simulink model "sampleModel7424_pp"  (R2018a)
settings: Solver=VariableStepAuto  StartTime=0.0  StopTime=10.0  RelTol=1e-3
undefined symbols (not defined in the file): DiscIntNeverNeededParam
libraries: simulink x211
(part 3 of 5)

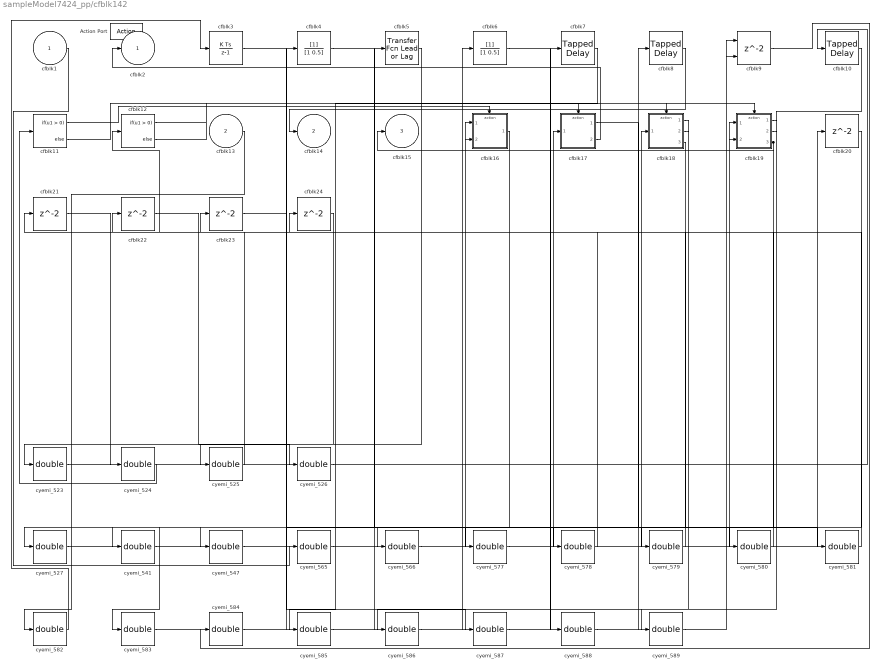
== system sampleModel7424_pp/cfblk142 ==
  cfblk1 : Inport
  cfblk13 : Inport  Port=2
  Action Port : ActionPort  ActionType=else
  cfblk10 : simulink/Discrete/Tapped Delay  vinit=0.0  samptime=-1  NumDelays=1  DelayOrder=Oldest  includeCurrent=off
  cfblk11 : If  SampleTime=1
  cfblk12 : If  SampleTime=1
  cfblk16 : Subsystem  TreatAsAtomicUnit=on
  cfblk17 : Subsystem  TreatAsAtomicUnit=on
  cfblk18 : Subsystem  TreatAsAtomicUnit=on
  cfblk19 : Subsystem  TreatAsAtomicUnit=on
  cfblk{20..24} (5 alike) : Delay
  cfblk3 : DiscreteIntegrator  SampleTime=-1  OutDataTypeStr=double  ICPrevOutput=DiscIntNeverNeededParam  ICPrevScaledInput=DiscIntNeverNeededParam
  cfblk4 : DiscreteFilter
  cfblk5 : simulink/Discrete/Transfer Fcn Lead or Lag  PoleZ=0.95  ZeroZ=0.75  ICPrevOutput=0.0  ICPrevInput=0.0  DoSatur=off
      settings: SourceProductName=Simulink  SourceProductBaseCode=SL
  cfblk6 : DiscreteFilter
  cfblk7 : simulink/Discrete/Tapped Delay  vinit=0.0  samptime=-1  NumDelays=1  DelayOrder=Oldest  includeCurrent=off
  cfblk8 : simulink/Discrete/Tapped Delay  vinit=0.0  samptime=-1  NumDelays=1  DelayOrder=Oldest  includeCurrent=off
  cfblk9 : Delay  ShowEnablePort=on
      settings: InputPortMap=u0,e6
  cyemi_{523..527,541,547,565..566,577..589} (22 alike) : DataTypeConversion  OutDataTypeStr=double
  cfblk2 : Outport
  cfblk14 : Outport  Port=2
  cfblk15 : Outport  Port=3
  wires:
  cfblk8/1 -> cfblk14/1
  cfblk19/3(cfblk13) -> cfblk15/1, cyemi_582/1
  cfblk17/2(cfblk7) -> cfblk2/1
  cfblk11/1 -> cfblk16/Action
  cfblk11/2 -> cfblk17/Action
  cfblk12/1 -> cfblk18/Action
  cfblk12/2 -> cfblk19/Action
  cyemi_523/1 -> cfblk10/1
  cfblk5/1 -> cyemi_523/1
  cyemi_524/1 -> cfblk11/1
  cfblk21/1 -> cyemi_524/1
  cyemi_525/1 -> cfblk12/1
  cfblk24/1 -> cyemi_525/1
  cyemi_526/1 -> cfblk16/1(cfblk1)
  cfblk22/1 -> cyemi_526/1
  cyemi_527/1 -> cfblk16/2(cfblk11)
  cfblk13/1 -> cyemi_527/1
  cyemi_541/1 -> cfblk17/1(cfblk1)
  cfblk19/1(cfblk2) -> cyemi_541/1
  cyemi_547/1 -> cfblk18/1(cfblk1)
  cfblk20/1 -> cyemi_547/1
  cyemi_565/1 -> cfblk19/1(cfblk1)
  cfblk1/1 -> cyemi_565/1
  cyemi_566/1 -> cfblk19/2(cfblk11)
  cfblk23/1 -> cyemi_566/1
  cyemi_577/1 -> cfblk20/1
  cfblk16/1(cfblk2) -> cyemi_577/1
  cyemi_578/1 -> cfblk21/1
  cfblk10/1 -> cyemi_578/1
  cyemi_579/1 -> cfblk22/1
  cfblk18/2(cfblk14) -> cyemi_579/1
  cyemi_580/1 -> cfblk23/1
  cfblk4/1 -> cyemi_580/1
  cyemi_581/1 -> cfblk24/1
  cfblk17/1(cfblk2) -> cyemi_581/1
  cyemi_582/1 -> cfblk3/1
  cyemi_583/1 -> cfblk4/1
  cfblk18/3(cfblk15) -> cyemi_583/1
  cyemi_584/1 -> cfblk5/1
  cfblk9/1 -> cyemi_584/1
  cyemi_585/1 -> cfblk6/1
  cfblk7/1 -> cyemi_585/1
  cyemi_586/1 -> cfblk7/1
  cfblk19/2(cfblk12) -> cyemi_586/1
  cyemi_587/1 -> cfblk8/1
  cfblk3/1 -> cyemi_587/1
  cyemi_588/1 -> cfblk9/1
  cfblk6/1 -> cyemi_588/1
  cyemi_589/1 -> cfblk9/2
  cfblk18/1(cfblk2) -> cyemi_589/1

== system sampleModel7424_pp/cfblk143 ==
  cfblk1 : Inport
  Action Port : ActionPort  ActionType=then
  cfblk3 : UnitDelay  SampleTime=-1
  cfblk4 : DiscreteZeroPole  Poles=[0 0.5]  Gain=1  SampleTime=-1
  cfblk5 : DiscreteZeroPole  Poles=[0 0.5]  Gain=1  SampleTime=-1
  cfblk6 : simulink/Discrete/Transfer Fcn First Order  PoleZ=0.95  ICPrevOutput=0.0  DoSatur=off
      settings: SourceProductName=Simulink
  cfblk7 : DiscreteZeroPole  Poles=[0 0.5]  Gain=1  SampleTime=-1
  cfblk8 : Delay
  cfblk9 : DataTypeConversion  OutDataTypeStr=double
  cyemi_{591..596} (6 alike) : DataTypeConversion  OutDataTypeStr=double
  cyemi_597 : DataTypeConversion  OutDataTypeStr=uint16
  cfblk2 : Outport
  wires:
  cfblk7/1 -> cfblk2/1
  cyemi_591/1 -> cfblk3/1
  cfblk8/1 -> cyemi_591/1
  cyemi_592/1 -> cfblk4/1
  cfblk6/1 -> cyemi_592/1
  cyemi_593/1 -> cfblk5/1
  cfblk4/1 -> cyemi_593/1
  cyemi_594/1 -> cfblk6/1
  cfblk3/1 -> cyemi_594/1
  cyemi_595/1 -> cfblk7/1
  cfblk9/1 -> cyemi_595/1
  cyemi_596/1 -> cfblk8/1
  cfblk5/1 -> cyemi_596/1
  cyemi_597/1 -> cfblk9/1
  cfblk1/1 -> cyemi_597/1

== system sampleModel7424_pp/cfblk144 ==
  cfblk1 : Inport
  cfblk12 : Inport  Port=2
  cfblk13 : Inport  Port=3
  Action Port : ActionPort  ActionType=else
  cfblk10 : simulink/Continuous/PID Controller  Controller=PID  TimeDomain=Discrete-time  SampleTime=-1  IntegratorMethod=Forward Euler  FilterMethod=Forward Euler  Form=Parallel  UseFilter=on  ControllerParametersSource=internal  P=1  I=1  D=0  N=100  InitialConditionSource=internal  InitialConditionForIntegrator=0  InitialConditionForFilter=0  ExternalReset=none  LimitOutput=off  UpperSaturationLimit=inf  LowerSaturationLimit=-inf  LinearizeAsGain=off  AntiWindupMode=none  Kb=1  TrackingMode=off  Kt=1  PParamMin=[]  PParamMax=[]  IParamMin=[]  IParamMax=[]  DParamMin=[]  DParamMax=[]  NParamMin=[]  NParamMax=[]  KbParamMin=[]  KbParamMax=[]  KtParamMin=[]  KtParamMax=[]  POutMin=[]  POutMax=[]  IOutMin=[]  IOutMax=[]  DOutMin=[]  DOutMax=[]  NOutMin=[]  NOutMax=[]  KbOutMin=[]  KbOutMax=[]  KtOutMin=[]  KtOutMax=[]  IntegratorOutMin=[]  IntegratorOutMax=[]  FilterOutMin=[]  FilterOutMax=[]  SumOutMin=[]  SumOutMax=[]  SumI1OutMin=[]  SumI1OutMax=[]  SumI2OutMin=[]  SumI2OutMax=[]  SumI3OutMin=[]  SumI3OutMax=[]  SumDOutMin=[]  SumDOutMax=[]  SaturationOutMin=[]  SaturationOutMax=[]  IntegratorContinuousStateAttributes=''  IntegratorStateMustResolveToSignalObject=off  IntegratorRTWStateStorageClass=Auto  FilterContinuousStateAttributes=''  FilterStateMustResolveToSignalObject=off  FilterRTWStateStorageClass=Auto  DifferentiatorICPrevScaledInput=0  DifferentiatorOutMin=[]  DifferentiatorOutMax=[]  FilterDiffOutCoefMin=[]  FilterDiffOutCoefMax=[]  SumDenOutMin=[]  SumDenOutMax=[]  SumNumOutMin=[]  SumNumOutMax=[]  ReciprocalOutMin=[]  ReciprocalOutMax=[]  DivideOutMin=[]  DivideOutMax=[]  TunerSelectOption=Transfer Function Based (PID Tuner App)
  cfblk11 : Delay  DelayLengthSource=Input port
      settings: InputPortMap=u0,p1
  cfblk14 : Delay
  cfblk3 : simulink/Discrete/Tapped Delay  vinit=0.0  samptime=-1  NumDelays=1  DelayOrder=Oldest  includeCurrent=off
  cfblk4 : simulink/Continuous/PID Controller  Controller=PID  TimeDomain=Discrete-time  SampleTime=-1  IntegratorMethod=Forward Euler  FilterMethod=Forward Euler  Form=Parallel  UseFilter=on  ControllerParametersSource=internal  P=1  I=1  D=0  N=100  InitialConditionSource=internal  InitialConditionForIntegrator=0  InitialConditionForFilter=0  ExternalReset=none  LimitOutput=off  UpperSaturationLimit=inf  LowerSaturationLimit=-inf  LinearizeAsGain=off  AntiWindupMode=none  Kb=1  TrackingMode=off  Kt=1  PParamMin=[]  PParamMax=[]  IParamMin=[]  IParamMax=[]  DParamMin=[]  DParamMax=[]  NParamMin=[]  NParamMax=[]  KbParamMin=[]  KbParamMax=[]  KtParamMin=[]  KtParamMax=[]  POutMin=[]  POutMax=[]  IOutMin=[]  IOutMax=[]  DOutMin=[]  DOutMax=[]  NOutMin=[]  NOutMax=[]  KbOutMin=[]  KbOutMax=[]  KtOutMin=[]  KtOutMax=[]  IntegratorOutMin=[]  IntegratorOutMax=[]  FilterOutMin=[]  FilterOutMax=[]  SumOutMin=[]  SumOutMax=[]  SumI1OutMin=[]  SumI1OutMax=[]  SumI2OutMin=[]  SumI2OutMax=[]  SumI3OutMin=[]  SumI3OutMax=[]  SumDOutMin=[]  SumDOutMax=[]  SaturationOutMin=[]  SaturationOutMax=[]  IntegratorContinuousStateAttributes=''  IntegratorStateMustResolveToSignalObject=off  IntegratorRTWStateStorageClass=Auto  FilterContinuousStateAttributes=''  FilterStateMustResolveToSignalObject=off  FilterRTWStateStorageClass=Auto  DifferentiatorICPrevScaledInput=0  DifferentiatorOutMin=[]  DifferentiatorOutMax=[]  FilterDiffOutCoefMin=[]  FilterDiffOutCoefMax=[]  SumDenOutMin=[]  SumDenOutMax=[]  SumNumOutMin=[]  SumNumOutMax=[]  ReciprocalOutMin=[]  ReciprocalOutMax=[]  DivideOutMin=[]  DivideOutMax=[]  TunerSelectOption=Transfer Function Based (PID Tuner App)
  cfblk5 : simulink/Discrete/Transfer Fcn Real Zero  ZeroZ=0.75  ICPrevInput=0.0  DoSatur=off
      settings: SourceProductName=Simulink  SourceProductBaseCode=SL
  cfblk6 : DiscreteFir
  cfblk7 : DiscreteFir
  cfblk8 : DiscreteTransferFcn
  cfblk9 : simulink/Discrete/Transfer Fcn Lead or Lag  PoleZ=0.95  ZeroZ=0.75  ICPrevOutput=0.0  ICPrevInput=0.0  DoSatur=off
      settings: SourceProductName=Simulink  SourceProductBaseCode=SL
  cyemi_{601..611} (11 alike) : DataTypeConversion  OutDataTypeStr=double
  cfblk2 : Outport
  wires:
  cfblk12/1 -> cfblk2/1
  cyemi_601/1 -> cfblk10/1
  cfblk5/1 -> cyemi_601/1
  cyemi_602/1 -> cfblk11/1
  cfblk1/1 -> cyemi_602/1
  cyemi_603/1 -> cfblk11/2
  cfblk3/1 -> cyemi_603/1
  cyemi_604/1 -> cfblk14/1
  cfblk7/1 -> cyemi_604/1
  cyemi_605/1 -> cfblk3/1
  cfblk9/1 -> cyemi_605/1
  cyemi_606/1 -> cfblk4/1
  cfblk13/1 -> cyemi_606/1
  cyemi_607/1 -> cfblk5/1
  cfblk4/1 -> cyemi_607/1
  cyemi_608/1 -> cfblk6/1
  cfblk14/1 -> cyemi_608/1
  cyemi_609/1 -> cfblk7/1
  cfblk8/1 -> cyemi_609/1
  cyemi_610/1 -> cfblk8/1
  cfblk6/1 -> cyemi_610/1
  cyemi_611/1 -> cfblk9/1
  cfblk10/1 -> cyemi_611/1

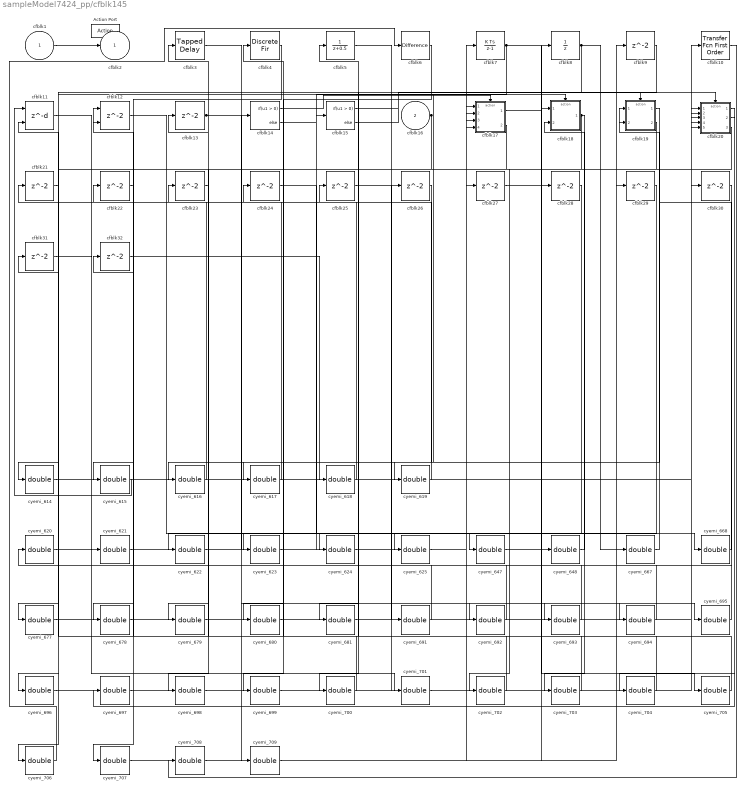
== system sampleModel7424_pp/cfblk145 ==
  cfblk1 : Inport
  cfblk16 : Inport  Port=2
  Action Port : ActionPort  ActionType=then
  cfblk10 : simulink/Discrete/Transfer Fcn First Order  PoleZ=0.95  ICPrevOutput=0.0  DoSatur=off
      settings: SourceProductName=Simulink
  cfblk11 : Delay  DelayLengthSource=Input port
      settings: InputPortMap=u0,p1
  cfblk12 : Delay  ShowEnablePort=on
      settings: InputPortMap=u0,e6
  cfblk{9,13,21..32} (14 alike) : Delay
  cfblk14 : If  SampleTime=1
  cfblk15 : If  SampleTime=1
  cfblk17 : Subsystem  TreatAsAtomicUnit=on
  cfblk18 : Subsystem  TreatAsAtomicUnit=on
  cfblk19 : Subsystem  TreatAsAtomicUnit=on
  cfblk20 : Subsystem  TreatAsAtomicUnit=on
  cfblk3 : simulink/Discrete/Tapped Delay  vinit=0.0  samptime=-1  NumDelays=1  DelayOrder=Oldest  includeCurrent=off
  cfblk4 : DiscreteFir
  cfblk5 : DiscreteTransferFcn
  cfblk6 : simulink/Discrete/Difference  ICPrevInput=0.0  OutMin=[]  OutMax=[]  OutDataTypeStr=double  OutputDataTypeScalingMode=double  OutDataType=fixdt(1, 16)  OutScaling=2^-10  DoSatur=off
  cfblk7 : DiscreteIntegrator  SampleTime=-1  OutDataTypeStr=double  ICPrevOutput=DiscIntNeverNeededParam  ICPrevScaledInput=DiscIntNeverNeededParam
  cfblk8 : UnitDelay  SampleTime=-1
  cyemi_{614..625,647..648,667..668,677..681,691..709} (40 alike) : DataTypeConversion  OutDataTypeStr=double
  cfblk2 : Outport
  wires:
  cfblk1/1 -> cfblk2/1
  cfblk8/1 -> cyemi_667/1, cyemi_681/1
  cfblk16/1 -> cyemi_615/1, cyemi_680/1
  cfblk13/1 -> cyemi_692/1, cyemi_693/1, cyemi_694/1
  cfblk7/1 -> cyemi_619/1, cyemi_695/1, cyemi_696/1
  cfblk18/1(cfblk2) -> cyemi_614/1, cyemi_624/1, cyemi_703/1
  cfblk14/1 -> cfblk17/Action
  cfblk14/2 -> cfblk18/Action
  cfblk15/1 -> cfblk19/Action
  cfblk15/2 -> cfblk20/Action
  cyemi_614/1 -> cfblk10/1
  cyemi_615/1 -> cfblk11/1
  cyemi_616/1 -> cfblk11/2
  cfblk19/1(cfblk2) -> cyemi_616/1
  cyemi_617/1 -> cfblk12/1
  cfblk6/1 -> cyemi_617/1
  cyemi_618/1 -> cfblk12/2
  cfblk32/1 -> cyemi_618/1
  cyemi_619/1 -> cfblk13/1
  cyemi_620/1 -> cfblk14/1
  cfblk30/1 -> cyemi_620/1
  cyemi_621/1 -> cfblk15/1
  cfblk31/1 -> cyemi_621/1
  cyemi_622/1 -> cfblk17/1(cfblk1)
  cfblk28/1 -> cyemi_622/1
  cyemi_623/1 -> cfblk17/2(cfblk14)
  cfblk26/1 -> cyemi_623/1
  cyemi_624/1 -> cfblk17/3(cfblk15)
  cyemi_625/1 -> cfblk17/4(cfblk16)
  cfblk24/1 -> cyemi_625/1
  cyemi_647/1 -> cfblk18/1(cfblk1)
  cfblk12/1 -> cyemi_647/1
  cyemi_648/1 -> cfblk18/2(cfblk15)
  cfblk27/1 -> cyemi_648/1
  cyemi_667/1 -> cfblk19/1(cfblk1)
  cyemi_668/1 -> cfblk19/2(cfblk11)
  cfblk25/1 -> cyemi_668/1
  cyemi_677/1 -> cfblk20/1(cfblk1)
  cfblk21/1 -> cyemi_677/1
  cyemi_678/1 -> cfblk20/2(cfblk10)
  cfblk22/1 -> cyemi_678/1
  cyemi_679/1 -> cfblk20/3(cfblk11)
  cfblk23/1 -> cyemi_679/1
  cyemi_680/1 -> cfblk20/4(cfblk12)
  cyemi_681/1 -> cfblk20/5(cfblk13)
  cyemi_691/1 -> cfblk21/1
  cfblk5/1 -> cyemi_691/1
  cyemi_692/1 -> cfblk22/1
  cyemi_693/1 -> cfblk23/1
  cyemi_694/1 -> cfblk24/1
  cyemi_695/1 -> cfblk25/1
  cyemi_696/1 -> cfblk26/1
  cyemi_697/1 -> cfblk27/1
  cfblk20/2(cfblk14) -> cyemi_697/1
  cyemi_698/1 -> cfblk28/1
  cfblk20/3(cfblk15) -> cyemi_698/1
  cyemi_699/1 -> cfblk29/1
  cfblk17/2(cfblk17) -> cyemi_699/1
  cyemi_700/1 -> cfblk3/1
  cfblk29/1 -> cyemi_700/1
  cyemi_701/1 -> cfblk30/1
  cfblk11/1 -> cyemi_701/1
  cyemi_702/1 -> cfblk31/1
  cfblk19/2(cfblk12) -> cyemi_702/1
  cyemi_703/1 -> cfblk32/1
  cyemi_704/1 -> cfblk4/1
  cfblk20/1(cfblk2) -> cyemi_704/1
  cyemi_705/1 -> cfblk5/1
  cfblk17/1(cfblk2) -> cyemi_705/1
  cyemi_706/1 -> cfblk6/1
  cfblk9/1 -> cyemi_706/1
  cyemi_707/1 -> cfblk7/1
  cfblk4/1 -> cyemi_707/1
  cyemi_708/1 -> cfblk8/1
  cfblk10/1 -> cyemi_708/1
  cyemi_709/1 -> cfblk9/1
  cfblk3/1 -> cyemi_709/1

== system sampleModel7424_pp/cfblk146 ==
  cfblk1 : Inport
  cfblk10 : Inport  Port=2
  Action Port : ActionPort  ActionType=else
  cfblk3 : UnitDelay  SampleTime=-1
  cfblk4 : DiscreteFilter
  cfblk5 : DiscreteZeroPole  Poles=[0 0.5]  Gain=1  SampleTime=-1
  cfblk6 : simulink/Discrete/Difference  ICPrevInput=0.0  OutMin=[]  OutMax=[]  OutDataTypeStr=double  OutputDataTypeScalingMode=double  OutDataType=fixdt(1, 16)  OutScaling=2^-10  DoSatur=off
  cfblk7 : simulink/Discrete/Difference  ICPrevInput=0.0  OutMin=[]  OutMax=[]  OutDataTypeStr=double  OutputDataTypeScalingMode=double  OutDataType=fixdt(1, 16)  OutScaling=2^-10  DoSatur=off
  cfblk8 : DiscreteFir
  cfblk9 : simulink/Continuous/PID Controller (2DOF)  Controller=PID  TimeDomain=Discrete-time  SampleTime=-1  IntegratorMethod=Forward Euler  FilterMethod=Forward Euler  Form=Parallel  UseFilter=on  ControllerParametersSource=internal  P=1  I=1  D=0  N=100  b=1  c=1  InitialConditionSource=internal  InitialConditionForIntegrator=0  InitialConditionForFilter=0  ExternalReset=none  LimitOutput=off  UpperSaturationLimit=inf  LowerSaturationLimit=-inf  LinearizeAsGain=off  AntiWindupMode=none  Kb=1  TrackingMode=off  Kt=1  PParamMin=[]  PParamMax=[]  IParamMin=[]  IParamMax=[]  DParamMin=[]  DParamMax=[]  NParamMin=[]  NParamMax=[]  bParamMin=[]  bParamMax=[]  cParamMin=[]  cParamMax=[]  KbParamMin=[]  KbParamMax=[]  KtParamMin=[]  KtParamMax=[]  POutMin=[]  POutMax=[]  IOutMin=[]  IOutMax=[]  DOutMin=[]  DOutMax=[]  NOutMin=[]  NOutMax=[]  bOutMin=[]  bOutMax=[]  cOutMin=[]  cOutMax=[]  KbOutMin=[]  KbOutMax=[]  KtOutMin=[]  KtOutMax=[]  IntegratorOutMin=[]  IntegratorOutMax=[]  FilterOutMin=[]  FilterOutMax=[]  SumOutMin=[]  SumOutMax=[]  Sum1OutMin=[]  Sum1OutMax=[]  Sum2OutMin=[]  Sum2OutMax=[]  Sum3OutMin=[]  Sum3OutMax=[]  SumI1OutMin=[]  SumI1OutMax=[]  SumI2OutMin=[]  SumI2OutMax=[]  SumI3OutMin=[]  SumI3OutMax=[]  SumDOutMin=[]  SumDOutMax=[]  SaturationOutMin=[]  SaturationOutMax=[]  IntegratorContinuousStateAttributes=''  IntegratorStateMustResolveToSignalObject=off  IntegratorRTWStateStorageClass=Auto  FilterContinuousStateAttributes=''  FilterStateMustResolveToSignalObject=off  FilterRTWStateStorageClass=Auto  DifferentiatorICPrevScaledInput=0  DifferentiatorOutMin=[]  DifferentiatorOutMax=[]  FilterDiffOutCoefMin=[]  FilterDiffOutCoefMax=[]  SumDenOutMin=[]  SumDenOutMax=[]  SumNumOutMin=[]  SumNumOutMax=[]  ReciprocalOutMin=[]  ReciprocalOutMax=[]  DivideOutMin=[]  DivideOutMax=[]  TunerSelectOption=Transfer Function Based (PID Tuner App)
  cyemi_{712..719} (8 alike) : DataTypeConversion  OutDataTypeStr=double
  cfblk2 : Outport
  cfblk11 : Outport  Port=2
  cfblk12 : Outport  Port=3
  wires:
  cfblk8/1 -> cfblk2/1
  cfblk4/1 -> cyemi_714/1, cyemi_719/1
  cfblk9/1 -> cfblk11/1
  cfblk6/1 -> cfblk12/1
  cfblk5/1 -> cyemi_712/1, cyemi_718/1
  cyemi_712/1 -> cfblk3/1
  cyemi_713/1 -> cfblk4/1
  cfblk10/1 -> cyemi_713/1
  cyemi_714/1 -> cfblk5/1
  cyemi_715/1 -> cfblk6/1
  cfblk7/1 -> cyemi_715/1
  cyemi_716/1 -> cfblk7/1
  cfblk3/1 -> cyemi_716/1
  cyemi_717/1 -> cfblk8/1
  cfblk1/1 -> cyemi_717/1
  cyemi_718/1 -> cfblk9/1
  cyemi_719/1 -> cfblk9/2

== system sampleModel7424_pp/cfblk147 ==
  cfblk1 : Inport
  cfblk10 : Inport  Port=2
  cfblk11 : Inport  Port=3
  Action Port : ActionPort  ActionType=then
  cfblk13 : Delay
  cfblk3 : DiscreteZeroPole  Poles=[0 0.5]  Gain=1  SampleTime=-1
  cfblk4 : Delay  DelayLengthSource=Input port
      settings: InputPortMap=u0,p1
  cfblk5 : DiscreteFilter
  cfblk6 : simulink/Discrete/Transfer Fcn First Order  PoleZ=0.95  ICPrevOutput=0.0  DoSatur=off
      settings: SourceProductName=Simulink
  cfblk7 : DiscreteFilter
  cfblk8 : DiscreteFilter
  cfblk9 : simulink/Discrete/Transfer Fcn Lead or Lag  PoleZ=0.95  ZeroZ=0.75  ICPrevOutput=0.0  ICPrevInput=0.0  DoSatur=off
      settings: SourceProductName=Simulink  SourceProductBaseCode=SL
  cyemi_{723..731} (9 alike) : DataTypeConversion  OutDataTypeStr=double
  cfblk2 : Outport
  cfblk12 : Outport  Port=2
  wires:
  cfblk3/1 -> cfblk2/1
  cfblk7/1 -> cfblk12/1
  cyemi_723/1 -> cfblk13/1
  cfblk8/1 -> cyemi_723/1
  cyemi_724/1 -> cfblk3/1
  cfblk5/1 -> cyemi_724/1
  cyemi_725/1 -> cfblk4/1
  cfblk13/1 -> cyemi_725/1
  cyemi_726/1 -> cfblk4/2
  cfblk9/1 -> cyemi_726/1
  cyemi_727/1 -> cfblk5/1
  cfblk10/1 -> cyemi_727/1
  cyemi_728/1 -> cfblk6/1
  cfblk4/1 -> cyemi_728/1
  cyemi_729/1 -> cfblk7/1
  cfblk11/1 -> cyemi_729/1
  cyemi_730/1 -> cfblk8/1
  cfblk6/1 -> cyemi_730/1
  cyemi_731/1 -> cfblk9/1
  cfblk1/1 -> cyemi_731/1

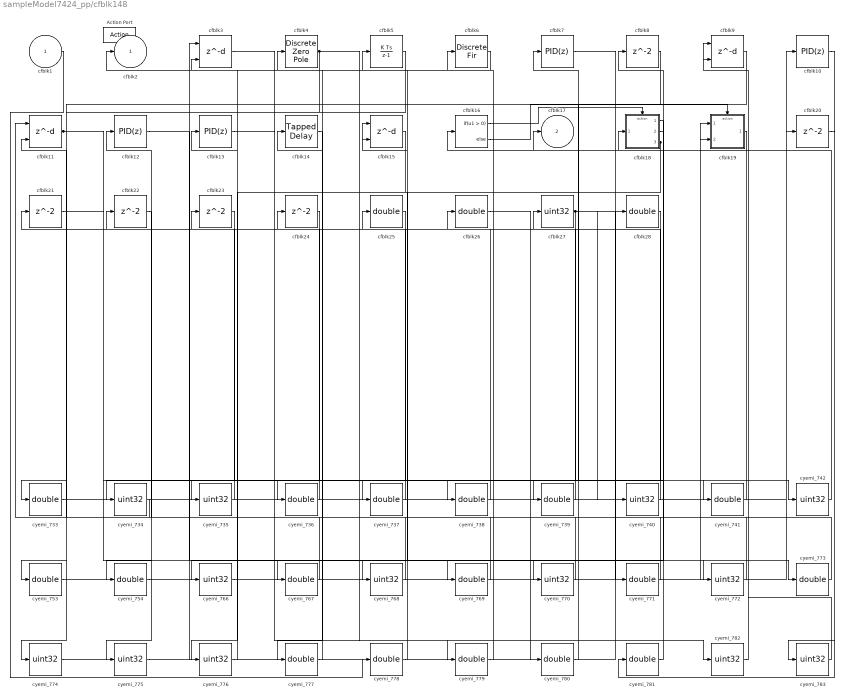
== system sampleModel7424_pp/cfblk148 ==
  cfblk1 : Inport
  Action Port : ActionPort  ActionType=else
  cfblk{7,10,12..13} (4 alike) : simulink/Continuous/PID Controller  Controller=PID  TimeDomain=Discrete-time  SampleTime=-1  IntegratorMethod=Forward Euler  FilterMethod=Forward Euler  Form=Parallel  UseFilter=on  ControllerParametersSource=internal  P=1  I=1  D=0  N=100  InitialConditionSource=internal  InitialConditionForIntegrator=0  InitialConditionForFilter=0  ExternalReset=none  LimitOutput=off  UpperSaturationLimit=inf  LowerSaturationLimit=-inf  LinearizeAsGain=off  AntiWindupMode=none  Kb=1  TrackingMode=off  Kt=1  PParamMin=[]  PParamMax=[]  IParamMin=[]  IParamMax=[]  DParamMin=[]  DParamMax=[]  NParamMin=[]  NParamMax=[]  KbParamMin=[]  KbParamMax=[]  KtParamMin=[]  KtParamMax=[]  POutMin=[]  POutMax=[]  IOutMin=[]  IOutMax=[]  DOutMin=[]  DOutMax=[]  NOutMin=[]  NOutMax=[]  KbOutMin=[]  KbOutMax=[]  KtOutMin=[]  KtOutMax=[]  IntegratorOutMin=[]  IntegratorOutMax=[]  FilterOutMin=[]  FilterOutMax=[]  SumOutMin=[]  SumOutMax=[]  SumI1OutMin=[]  SumI1OutMax=[]  SumI2OutMin=[]  SumI2OutMax=[]  SumI3OutMin=[]  SumI3OutMax=[]  SumDOutMin=[]  SumDOutMax=[]  SaturationOutMin=[]  SaturationOutMax=[]  IntegratorContinuousStateAttributes=''  IntegratorStateMustResolveToSignalObject=off  IntegratorRTWStateStorageClass=Auto  FilterContinuousStateAttributes=''  FilterStateMustResolveToSignalObject=off  FilterRTWStateStorageClass=Auto  DifferentiatorICPrevScaledInput=0  DifferentiatorOutMin=[]  DifferentiatorOutMax=[]  FilterDiffOutCoefMin=[]  FilterDiffOutCoefMax=[]  SumDenOutMin=[]  SumDenOutMax=[]  SumNumOutMin=[]  SumNumOutMax=[]  ReciprocalOutMin=[]  ReciprocalOutMax=[]  DivideOutMin=[]  DivideOutMax=[]  TunerSelectOption=Transfer Function Based (PID Tuner App)
  cfblk{3,9,11,15} (4 alike) : Delay  DelayLengthSource=Input port
      settings: InputPortMap=u0,p1
  cfblk14 : simulink/Discrete/Tapped Delay  vinit=0.0  samptime=-1  NumDelays=1  DelayOrder=Oldest  includeCurrent=off
  cfblk16 : If  SampleTime=1
  cfblk18 : Subsystem  TreatAsAtomicUnit=on
  cfblk19 : Subsystem  TreatAsAtomicUnit=on
  cfblk{8,20..24} (6 alike) : Delay
  cfblk25 : DataTypeConversion  OutDataTypeStr=double
  cfblk26 : DataTypeConversion  OutDataTypeStr=double
  cfblk27 : DataTypeConversion  OutDataTypeStr=uint32
  cfblk28 : DataTypeConversion  OutDataTypeStr=double
  cfblk4 : DiscreteZeroPole  Poles=[0 0.5]  Gain=1  SampleTime=-1
  cfblk5 : DiscreteIntegrator  SampleTime=-1  OutDataTypeStr=double  ICPrevOutput=DiscIntNeverNeededParam  ICPrevScaledInput=DiscIntNeverNeededParam
  cfblk6 : DiscreteFir
  cyemi_{733,736..739,741,753..754,767,769,771,773,777..781} (17 alike) : DataTypeConversion  OutDataTypeStr=double
  cyemi_{734..735,740,742,766,768,770,772,774..776,782..783} (13 alike) : DataTypeConversion  OutDataTypeStr=uint32
  cfblk2 : Outport
  cfblk17 : Outport  Port=2
  wires:
  cfblk4/1 -> cyemi_753/1, cyemi_779/1
  cfblk11/1 -> cyemi_770/1, cyemi_772/1
  cfblk6/1 -> cfblk2/1
  cfblk19/1(cfblk2) -> cfblk17/1
  cfblk18/3(cfblk10) -> cyemi_735/1, cyemi_768/1
  cfblk16/1 -> cfblk18/Action
  cfblk16/2 -> cfblk19/Action
  cfblk27/1 -> cyemi_734/1, cyemi_740/1, cyemi_742/1
  cyemi_733/1 -> cfblk10/1
  cfblk5/1 -> cyemi_733/1
  cyemi_734/1 -> cfblk11/1
  cyemi_735/1 -> cfblk11/2
  cyemi_736/1 -> cfblk12/1
  cfblk25/1 -> cyemi_736/1
  cyemi_737/1 -> cfblk13/1
  cfblk28/1 -> cyemi_737/1
  cyemi_738/1 -> cfblk14/1
  cfblk18/2(cfblk9) -> cyemi_738/1
  cyemi_739/1 -> cfblk15/1
  cfblk8/1 -> cyemi_739/1
  cyemi_740/1 -> cfblk15/2
  cyemi_741/1 -> cfblk16/1
  cfblk21/1 -> cyemi_741/1
  cyemi_742/1 -> cfblk18/1(cfblk1)
  cyemi_753/1 -> cfblk19/1(cfblk1)
  cyemi_754/1 -> cfblk19/2(cfblk11)
  cfblk23/1 -> cyemi_754/1
  cyemi_766/1 -> cfblk20/1
  cfblk18/1(cfblk2) -> cyemi_766/1
  cyemi_767/1 -> cfblk21/1
  cfblk14/1 -> cyemi_767/1
  cyemi_768/1 -> cfblk22/1
  cyemi_769/1 -> cfblk23/1
  cfblk12/1 -> cyemi_769/1
  cyemi_770/1 -> cfblk24/1
  cyemi_771/1 -> cfblk25/1
  cfblk7/1 -> cyemi_771/1
  cyemi_772/1 -> cfblk26/1
  cyemi_773/1 -> cfblk27/1
  cfblk13/1 -> cyemi_773/1
  cyemi_774/1 -> cfblk28/1
  cfblk9/1 -> cyemi_774/1
  cyemi_775/1 -> cfblk3/1
  cfblk22/1 -> cyemi_775/1
  cyemi_776/1 -> cfblk3/2
  cfblk24/1 -> cyemi_776/1
  cyemi_777/1 -> cfblk4/1
  cfblk15/1 -> cyemi_777/1
  cyemi_778/1 -> cfblk5/1
  cfblk1/1 -> cyemi_778/1
  cyemi_779/1 -> cfblk6/1
  cyemi_780/1 -> cfblk7/1
  cfblk26/1 -> cyemi_780/1
  cyemi_781/1 -> cfblk8/1
  cfblk10/1 -> cyemi_781/1
  cyemi_782/1 -> cfblk9/1
  cfblk3/1 -> cyemi_782/1
  cyemi_783/1 -> cfblk9/2
  cfblk20/1 -> cyemi_783/1

== system sampleModel7424_pp/cfblk124/cfblk14 ==
  cfblk1 : Inport
  Action Port : ActionPort  ActionType=then
  cfblk3 : DiscreteFilter
  cfblk4 : DiscreteZeroPole  Poles=[0 0.5]  Gain=1  SampleTime=-1
  cfblk5 : UnitDelay  SampleTime=-1
  cfblk6 : DiscreteZeroPole  Poles=[0 0.5]  Gain=1  SampleTime=-1
  cyemi_{33..36} (4 alike) : DataTypeConversion  OutDataTypeStr=double
  cfblk2 : Outport
  cfblk7 : Outport  Port=2
  wires:
  cfblk1/1 -> cyemi_33/1, cyemi_36/1
  cfblk6/1 -> cfblk7/1
  cfblk4/1 -> cfblk2/1
  cyemi_33/1 -> cfblk3/1
  cyemi_34/1 -> cfblk4/1
  cfblk5/1 -> cyemi_34/1
  cyemi_35/1 -> cfblk5/1
  cfblk3/1 -> cyemi_35/1
  cyemi_36/1 -> cfblk6/1

== system sampleModel7424_pp/cfblk124/cfblk15 ==
  cfblk1 : Inport
  cfblk15 : Inport  Port=2
  cfblk16 : Inport  Port=3
  Action Port : ActionPort  ActionType=else
  cfblk10 : simulink/Discrete/Transfer Fcn Real Zero  ZeroZ=0.75  ICPrevInput=0.0  DoSatur=off
      settings: SourceProductName=Simulink  SourceProductBaseCode=SL
  cfblk11 : simulink/Discrete/Transfer Fcn Lead or Lag  PoleZ=0.95  ZeroZ=0.75  ICPrevOutput=0.0  ICPrevInput=0.0  DoSatur=off
      settings: SourceProductName=Simulink  SourceProductBaseCode=SL
  cfblk12 : simulink/Discrete/Transfer Fcn First Order  PoleZ=0.95  ICPrevOutput=0.0  DoSatur=off
      settings: SourceProductName=Simulink
  cfblk13 : DiscreteFilter
  cfblk14 : simulink/Discrete/Difference  ICPrevInput=0.0  OutMin=[]  OutMax=[]  OutDataTypeStr=double  OutputDataTypeScalingMode=double  OutDataType=fixdt(1, 16)  OutScaling=2^-10  DoSatur=off
  cfblk17 : Delay
  cfblk18 : Delay
  cfblk3 : Delay  DelayLengthSource=Input port
      settings: InputPortMap=u0,p1
  cfblk4 : DiscreteStateSpace  SampleTime=-1
  cfblk5 : DiscreteIntegrator  SampleTime=-1  OutDataTypeStr=double  ICPrevOutput=DiscIntNeverNeededParam  ICPrevScaledInput=DiscIntNeverNeededParam
  cfblk6 : simulink/Discrete/Transfer Fcn Real Zero  ZeroZ=0.75  ICPrevInput=0.0  DoSatur=off
      settings: SourceProductName=Simulink  SourceProductBaseCode=SL
  cfblk7 : Delay  ShowEnablePort=on
      settings: InputPortMap=u0,e6
  cfblk8 : DiscreteFilter
  cfblk9 : simulink/Continuous/PID Controller  Controller=PID  TimeDomain=Discrete-time  SampleTime=-1  IntegratorMethod=Forward Euler  FilterMethod=Forward Euler  Form=Parallel  UseFilter=on  ControllerParametersSource=internal  P=1  I=1  D=0  N=100  InitialConditionSource=internal  InitialConditionForIntegrator=0  InitialConditionForFilter=0  ExternalReset=none  LimitOutput=off  UpperSaturationLimit=inf  LowerSaturationLimit=-inf  LinearizeAsGain=off  AntiWindupMode=none  Kb=1  TrackingMode=off  Kt=1  PParamMin=[]  PParamMax=[]  IParamMin=[]  IParamMax=[]  DParamMin=[]  DParamMax=[]  NParamMin=[]  NParamMax=[]  KbParamMin=[]  KbParamMax=[]  KtParamMin=[]  KtParamMax=[]  POutMin=[]  POutMax=[]  IOutMin=[]  IOutMax=[]  DOutMin=[]  DOutMax=[]  NOutMin=[]  NOutMax=[]  KbOutMin=[]  KbOutMax=[]  KtOutMin=[]  KtOutMax=[]  IntegratorOutMin=[]  IntegratorOutMax=[]  FilterOutMin=[]  FilterOutMax=[]  SumOutMin=[]  SumOutMax=[]  SumI1OutMin=[]  SumI1OutMax=[]  SumI2OutMin=[]  SumI2OutMax=[]  SumI3OutMin=[]  SumI3OutMax=[]  SumDOutMin=[]  SumDOutMax=[]  SaturationOutMin=[]  SaturationOutMax=[]  IntegratorContinuousStateAttributes=''  IntegratorStateMustResolveToSignalObject=off  IntegratorRTWStateStorageClass=Auto  FilterContinuousStateAttributes=''  FilterStateMustResolveToSignalObject=off  FilterRTWStateStorageClass=Auto  DifferentiatorICPrevScaledInput=0  DifferentiatorOutMin=[]  DifferentiatorOutMax=[]  FilterDiffOutCoefMin=[]  FilterDiffOutCoefMax=[]  SumDenOutMin=[]  SumDenOutMax=[]  SumNumOutMin=[]  SumNumOutMax=[]  ReciprocalOutMin=[]  ReciprocalOutMax=[]  DivideOutMin=[]  DivideOutMax=[]  TunerSelectOption=Transfer Function Based (PID Tuner App)
  cyemi_{40..55} (16 alike) : DataTypeConversion  OutDataTypeStr=double
  cfblk2 : Outport
  wires:
  cfblk1/1 -> cyemi_50/1, cyemi_51/1
  cfblk10/1 -> cfblk2/1
  cyemi_40/1 -> cfblk10/1
  cfblk3/1 -> cyemi_40/1
  cyemi_41/1 -> cfblk11/1
  cfblk13/1 -> cyemi_41/1
  cyemi_42/1 -> cfblk12/1
  cfblk11/1 -> cyemi_42/1
  cyemi_43/1 -> cfblk13/1
  cfblk15/1 -> cyemi_43/1
  cyemi_44/1 -> cfblk14/1
  cfblk8/1 -> cyemi_44/1
  cyemi_45/1 -> cfblk17/1
  cfblk7/1 -> cyemi_45/1
  cyemi_46/1 -> cfblk18/1
  cfblk14/1 -> cyemi_46/1
  cyemi_47/1 -> cfblk3/1
  cfblk5/1 -> cyemi_47/1
  cyemi_48/1 -> cfblk3/2
  cfblk12/1 -> cyemi_48/1
  cyemi_49/1 -> cfblk4/1
  cfblk17/1 -> cyemi_49/1
  cyemi_50/1 -> cfblk5/1
  cyemi_51/1 -> cfblk6/1
  cyemi_52/1 -> cfblk7/1
  cfblk4/1 -> cyemi_52/1
  cyemi_53/1 -> cfblk7/2
  cfblk9/1 -> cyemi_53/1
  cyemi_54/1 -> cfblk8/1
  cfblk18/1 -> cyemi_54/1
  cyemi_55/1 -> cfblk9/1
  cfblk16/1 -> cyemi_55/1

== system sampleModel7424_pp/cfblk124/cfblk16 ==
  cfblk1 : Inport
  cfblk11 : Inport  Port=2
  cfblk12 : Inport  Port=3
  cfblk13 : Inport  Port=4
  cfblk14 : Inport  Port=5
  Action Port : ActionPort  ActionType=then
  cfblk10 : simulink/Discrete/Transfer Fcn First Order  PoleZ=0.95  ICPrevOutput=0.0  DoSatur=off
      settings: SourceProductName=Simulink
  cfblk15 : Delay
  cfblk16 : Delay
  cfblk3 : DiscreteFir
  cfblk4 : Delay  DelayLengthSource=Input port
      settings: InputPortMap=u0,p1
  cfblk5 : DiscreteStateSpace  SampleTime=-1
  cfblk6 : simulink/Discrete/Transfer Fcn Real Zero  ZeroZ=0.75  ICPrevInput=0.0  DoSatur=off
      settings: SourceProductName=Simulink  SourceProductBaseCode=SL
  cfblk7 : Delay  ShowEnablePort=on
      settings: InputPortMap=u0,e6
  cfblk8 : simulink/Discrete/Transfer Fcn Real Zero  ZeroZ=0.75  ICPrevInput=0.0  DoSatur=off
      settings: SourceProductName=Simulink  SourceProductBaseCode=SL
  cfblk9 : Delay
  cyemi_{61..72} (12 alike) : DataTypeConversion  OutDataTypeStr=double
  cfblk2 : Outport
  wires:
  cfblk1/1 -> cfblk2/1
  cyemi_61/1 -> cfblk10/1
  cfblk13/1 -> cyemi_61/1
  cyemi_62/1 -> cfblk15/1
  cfblk7/1 -> cyemi_62/1
  cyemi_63/1 -> cfblk16/1
  cfblk6/1 -> cyemi_63/1
  cyemi_64/1 -> cfblk3/1
  cfblk12/1 -> cyemi_64/1
  cyemi_65/1 -> cfblk4/1
  cfblk14/1 -> cyemi_65/1
  cyemi_66/1 -> cfblk4/2
  cfblk15/1 -> cyemi_66/1
  cyemi_67/1 -> cfblk5/1
  cfblk16/1 -> cyemi_67/1
  cyemi_68/1 -> cfblk6/1
  cfblk5/1 -> cyemi_68/1
  cyemi_69/1 -> cfblk7/1
  cfblk11/1 -> cyemi_69/1
  cyemi_70/1 -> cfblk7/2
  cfblk9/1 -> cyemi_70/1
  cyemi_71/1 -> cfblk8/1
  cfblk10/1 -> cyemi_71/1
  cyemi_72/1 -> cfblk9/1
  cfblk4/1 -> cyemi_72/1

== system sampleModel7424_pp/cfblk124/cfblk17 ==
  cfblk1 : Inport
  cfblk12 : Inport  Port=2
  cfblk13 : Inport  Port=3
  cfblk14 : Inport  Port=4
  cfblk15 : Inport  Port=5
  Action Port : ActionPort  ActionType=else
  cfblk10 : DiscreteFilter
  cfblk11 : simulink/Discrete/Transfer Fcn Real Zero  ZeroZ=0.75  ICPrevInput=0.0  DoSatur=off
      settings: SourceProductName=Simulink  SourceProductBaseCode=SL
  cfblk16 : Delay
  cfblk3 : DiscreteFilter
  cfblk4 : DiscreteZeroPole  Poles=[0 0.5]  Gain=1  SampleTime=-1
  cfblk5 : simulink/Discrete/Transfer Fcn Real Zero  ZeroZ=0.75  ICPrevInput=0.0  DoSatur=off
      settings: SourceProductName=Simulink  SourceProductBaseCode=SL
  cfblk6 : UnitDelay  SampleTime=-1
  cfblk7 : simulink/Discrete/Transfer Fcn Real Zero  ZeroZ=0.75  ICPrevInput=0.0  DoSatur=off
      settings: SourceProductName=Simulink  SourceProductBaseCode=SL
  cfblk8 : DiscreteFir
  cfblk9 : simulink/Continuous/PID Controller  Controller=PID  TimeDomain=Discrete-time  SampleTime=-1  IntegratorMethod=Forward Euler  FilterMethod=Forward Euler  Form=Parallel  UseFilter=on  ControllerParametersSource=internal  P=1  I=1  D=0  N=100  InitialConditionSource=internal  InitialConditionForIntegrator=0  InitialConditionForFilter=0  ExternalReset=none  LimitOutput=off  UpperSaturationLimit=inf  LowerSaturationLimit=-inf  LinearizeAsGain=off  AntiWindupMode=none  Kb=1  TrackingMode=off  Kt=1  PParamMin=[]  PParamMax=[]  IParamMin=[]  IParamMax=[]  DParamMin=[]  DParamMax=[]  NParamMin=[]  NParamMax=[]  KbParamMin=[]  KbParamMax=[]  KtParamMin=[]  KtParamMax=[]  POutMin=[]  POutMax=[]  IOutMin=[]  IOutMax=[]  DOutMin=[]  DOutMax=[]  NOutMin=[]  NOutMax=[]  KbOutMin=[]  KbOutMax=[]  KtOutMin=[]  KtOutMax=[]  IntegratorOutMin=[]  IntegratorOutMax=[]  FilterOutMin=[]  FilterOutMax=[]  SumOutMin=[]  SumOutMax=[]  SumI1OutMin=[]  SumI1OutMax=[]  SumI2OutMin=[]  SumI2OutMax=[]  SumI3OutMin=[]  SumI3OutMax=[]  SumDOutMin=[]  SumDOutMax=[]  SaturationOutMin=[]  SaturationOutMax=[]  IntegratorContinuousStateAttributes=''  IntegratorStateMustResolveToSignalObject=off  IntegratorRTWStateStorageClass=Auto  FilterContinuousStateAttributes=''  FilterStateMustResolveToSignalObject=off  FilterRTWStateStorageClass=Auto  DifferentiatorICPrevScaledInput=0  DifferentiatorOutMin=[]  DifferentiatorOutMax=[]  FilterDiffOutCoefMin=[]  FilterDiffOutCoefMax=[]  SumDenOutMin=[]  SumDenOutMax=[]  SumNumOutMin=[]  SumNumOutMax=[]  ReciprocalOutMin=[]  ReciprocalOutMax=[]  DivideOutMin=[]  DivideOutMax=[]  TunerSelectOption=Transfer Function Based (PID Tuner App)
  cyemi_{78..87} (10 alike) : DataTypeConversion  OutDataTypeStr=double
  cfblk2 : Outport
  wires:
  cfblk3/1 -> cfblk2/1
  cyemi_78/1 -> cfblk10/1
  cfblk14/1 -> cyemi_78/1
  cyemi_79/1 -> cfblk11/1
  cfblk4/1 -> cyemi_79/1
  cyemi_80/1 -> cfblk16/1
  cfblk7/1 -> cyemi_80/1
  cyemi_81/1 -> cfblk3/1
  cfblk5/1 -> cyemi_81/1
  cyemi_82/1 -> cfblk4/1
  cfblk16/1 -> cyemi_82/1
  cyemi_83/1 -> cfblk5/1
  cfblk13/1 -> cyemi_83/1
  cyemi_84/1 -> cfblk6/1
  cfblk9/1 -> cyemi_84/1
  cyemi_85/1 -> cfblk7/1
  cfblk6/1 -> cyemi_85/1
  cyemi_86/1 -> cfblk8/1
  cfblk15/1 -> cyemi_86/1
  cyemi_87/1 -> cfblk9/1
  cfblk11/1 -> cyemi_87/1

== system sampleModel7424_pp/cfblk125/cfblk11 ==
  cfblk1 : Inport
  cfblk12 : Inport  Port=2
  Action Port : ActionPort  ActionType=then
  cfblk10 : DiscreteFilter
  cfblk11 : simulink/Discrete/Transfer Fcn Real Zero  ZeroZ=0.75  ICPrevInput=0.0  DoSatur=off
      settings: SourceProductName=Simulink  SourceProductBaseCode=SL
  cfblk15 : Delay
  cfblk16 : DataTypeConversion  OutDataTypeStr=uint32
  cfblk17 : DataTypeConversion  OutDataTypeStr=double
  cfblk3 : DiscreteFir
  cfblk4 : simulink/Continuous/PID Controller  Controller=PID  TimeDomain=Discrete-time  SampleTime=-1  IntegratorMethod=Forward Euler  FilterMethod=Forward Euler  Form=Parallel  UseFilter=on  ControllerParametersSource=internal  P=1  I=1  D=0  N=100  InitialConditionSource=internal  InitialConditionForIntegrator=0  InitialConditionForFilter=0  ExternalReset=none  LimitOutput=off  UpperSaturationLimit=inf  LowerSaturationLimit=-inf  LinearizeAsGain=off  AntiWindupMode=none  Kb=1  TrackingMode=off  Kt=1  PParamMin=[]  PParamMax=[]  IParamMin=[]  IParamMax=[]  DParamMin=[]  DParamMax=[]  NParamMin=[]  NParamMax=[]  KbParamMin=[]  KbParamMax=[]  KtParamMin=[]  KtParamMax=[]  POutMin=[]  POutMax=[]  IOutMin=[]  IOutMax=[]  DOutMin=[]  DOutMax=[]  NOutMin=[]  NOutMax=[]  KbOutMin=[]  KbOutMax=[]  KtOutMin=[]  KtOutMax=[]  IntegratorOutMin=[]  IntegratorOutMax=[]  FilterOutMin=[]  FilterOutMax=[]  SumOutMin=[]  SumOutMax=[]  SumI1OutMin=[]  SumI1OutMax=[]  SumI2OutMin=[]  SumI2OutMax=[]  SumI3OutMin=[]  SumI3OutMax=[]  SumDOutMin=[]  SumDOutMax=[]  SaturationOutMin=[]  SaturationOutMax=[]  IntegratorContinuousStateAttributes=''  IntegratorStateMustResolveToSignalObject=off  IntegratorRTWStateStorageClass=Auto  FilterContinuousStateAttributes=''  FilterStateMustResolveToSignalObject=off  FilterRTWStateStorageClass=Auto  DifferentiatorICPrevScaledInput=0  DifferentiatorOutMin=[]  DifferentiatorOutMax=[]  FilterDiffOutCoefMin=[]  FilterDiffOutCoefMax=[]  SumDenOutMin=[]  SumDenOutMax=[]  SumNumOutMin=[]  SumNumOutMax=[]  ReciprocalOutMin=[]  ReciprocalOutMax=[]  DivideOutMin=[]  DivideOutMax=[]  TunerSelectOption=Transfer Function Based (PID Tuner App)
  cfblk5 : DiscreteFir
  cfblk6 : Delay  DelayLengthSource=Input port
      settings: InputPortMap=u0,p1
  cfblk7 : DiscreteZeroPole  Poles=[0 0.5]  Gain=1  SampleTime=-1
  cfblk8 : simulink/Discrete/Tapped Delay  vinit=0.0  samptime=-1  NumDelays=1  DelayOrder=Oldest  includeCurrent=off
  cfblk9 : DiscreteFilter
  cyemi_{114..122,124..126} (12 alike) : DataTypeConversion  OutDataTypeStr=double
  cyemi_123 : DataTypeConversion  OutDataTypeStr=uint32
  cfblk2 : Outport
  cfblk13 : Outport  Port=2
  cfblk14 : Outport  Port=3
  wires:
  cfblk5/1 -> cfblk14/1
  cfblk4/1 -> cfblk13/1
  cfblk7/1 -> cfblk2/1, cyemi_115/1
  cfblk3/1 -> cyemi_118/1, cyemi_125/1
  cyemi_114/1 -> cfblk10/1
  cfblk17/1 -> cyemi_114/1
  cyemi_115/1 -> cfblk11/1
  cyemi_116/1 -> cfblk15/1
  cfblk9/1 -> cyemi_116/1
  cyemi_117/1 -> cfblk16/1
  cfblk10/1 -> cyemi_117/1
  cyemi_118/1 -> cfblk17/1
  cyemi_119/1 -> cfblk3/1
  cfblk15/1 -> cyemi_119/1
  cyemi_120/1 -> cfblk4/1
  cfblk1/1 -> cyemi_120/1
  cyemi_121/1 -> cfblk5/1
  cfblk6/1 -> cyemi_121/1
  cyemi_122/1 -> cfblk6/1
  cfblk11/1 -> cyemi_122/1
  cyemi_123/1 -> cfblk6/2
  cfblk16/1 -> cyemi_123/1
  cyemi_124/1 -> cfblk7/1
  cfblk12/1 -> cyemi_124/1
  cyemi_125/1 -> cfblk8/1
  cyemi_126/1 -> cfblk9/1
  cfblk8/1 -> cyemi_126/1

== system sampleModel7424_pp/cfblk125/cfblk12 ==
  cfblk1 : Inport
  Action Port : ActionPort  ActionType=else
  cfblk10 : simulink/Continuous/PID Controller  Controller=PID  TimeDomain=Discrete-time  SampleTime=-1  IntegratorMethod=Forward Euler  FilterMethod=Forward Euler  Form=Parallel  UseFilter=on  ControllerParametersSource=internal  P=1  I=1  D=0  N=100  InitialConditionSource=internal  InitialConditionForIntegrator=0  InitialConditionForFilter=0  ExternalReset=none  LimitOutput=off  UpperSaturationLimit=inf  LowerSaturationLimit=-inf  LinearizeAsGain=off  AntiWindupMode=none  Kb=1  TrackingMode=off  Kt=1  PParamMin=[]  PParamMax=[]  IParamMin=[]  IParamMax=[]  DParamMin=[]  DParamMax=[]  NParamMin=[]  NParamMax=[]  KbParamMin=[]  KbParamMax=[]  KtParamMin=[]  KtParamMax=[]  POutMin=[]  POutMax=[]  IOutMin=[]  IOutMax=[]  DOutMin=[]  DOutMax=[]  NOutMin=[]  NOutMax=[]  KbOutMin=[]  KbOutMax=[]  KtOutMin=[]  KtOutMax=[]  IntegratorOutMin=[]  IntegratorOutMax=[]  FilterOutMin=[]  FilterOutMax=[]  SumOutMin=[]  SumOutMax=[]  SumI1OutMin=[]  SumI1OutMax=[]  SumI2OutMin=[]  SumI2OutMax=[]  SumI3OutMin=[]  SumI3OutMax=[]  SumDOutMin=[]  SumDOutMax=[]  SaturationOutMin=[]  SaturationOutMax=[]  IntegratorContinuousStateAttributes=''  IntegratorStateMustResolveToSignalObject=off  IntegratorRTWStateStorageClass=Auto  FilterContinuousStateAttributes=''  FilterStateMustResolveToSignalObject=off  FilterRTWStateStorageClass=Auto  DifferentiatorICPrevScaledInput=0  DifferentiatorOutMin=[]  DifferentiatorOutMax=[]  FilterDiffOutCoefMin=[]  FilterDiffOutCoefMax=[]  SumDenOutMin=[]  SumDenOutMax=[]  SumNumOutMin=[]  SumNumOutMax=[]  ReciprocalOutMin=[]  ReciprocalOutMax=[]  DivideOutMin=[]  DivideOutMax=[]  TunerSelectOption=Transfer Function Based (PID Tuner App)
  cfblk11 : DiscreteFir
  cfblk12 : simulink/Continuous/PID Controller (2DOF)  Controller=PID  TimeDomain=Discrete-time  SampleTime=-1  IntegratorMethod=Forward Euler  FilterMethod=Forward Euler  Form=Parallel  UseFilter=on  ControllerParametersSource=internal  P=1  I=1  D=0  N=100  b=1  c=1  InitialConditionSource=internal  InitialConditionForIntegrator=0  InitialConditionForFilter=0  ExternalReset=none  LimitOutput=off  UpperSaturationLimit=inf  LowerSaturationLimit=-inf  LinearizeAsGain=off  AntiWindupMode=none  Kb=1  TrackingMode=off  Kt=1  PParamMin=[]  PParamMax=[]  IParamMin=[]  IParamMax=[]  DParamMin=[]  DParamMax=[]  NParamMin=[]  NParamMax=[]  bParamMin=[]  bParamMax=[]  cParamMin=[]  cParamMax=[]  KbParamMin=[]  KbParamMax=[]  KtParamMin=[]  KtParamMax=[]  POutMin=[]  POutMax=[]  IOutMin=[]  IOutMax=[]  DOutMin=[]  DOutMax=[]  NOutMin=[]  NOutMax=[]  bOutMin=[]  bOutMax=[]  cOutMin=[]  cOutMax=[]  KbOutMin=[]  KbOutMax=[]  KtOutMin=[]  KtOutMax=[]  IntegratorOutMin=[]  IntegratorOutMax=[]  FilterOutMin=[]  FilterOutMax=[]  SumOutMin=[]  SumOutMax=[]  Sum1OutMin=[]  Sum1OutMax=[]  Sum2OutMin=[]  Sum2OutMax=[]  Sum3OutMin=[]  Sum3OutMax=[]  SumI1OutMin=[]  SumI1OutMax=[]  SumI2OutMin=[]  SumI2OutMax=[]  SumI3OutMin=[]  SumI3OutMax=[]  SumDOutMin=[]  SumDOutMax=[]  SaturationOutMin=[]  SaturationOutMax=[]  IntegratorContinuousStateAttributes=''  IntegratorStateMustResolveToSignalObject=off  IntegratorRTWStateStorageClass=Auto  FilterContinuousStateAttributes=''  FilterStateMustResolveToSignalObject=off  FilterRTWStateStorageClass=Auto  DifferentiatorICPrevScaledInput=0  DifferentiatorOutMin=[]  DifferentiatorOutMax=[]  FilterDiffOutCoefMin=[]  FilterDiffOutCoefMax=[]  SumDenOutMin=[]  SumDenOutMax=[]  SumNumOutMin=[]  SumNumOutMax=[]  ReciprocalOutMin=[]  ReciprocalOutMax=[]  DivideOutMin=[]  DivideOutMax=[]  TunerSelectOption=Transfer Function Based (PID Tuner App)
  cfblk13 : simulink/Discrete/Transfer Fcn Lead or Lag  PoleZ=0.95  ZeroZ=0.75  ICPrevOutput=0.0  ICPrevInput=0.0  DoSatur=off
      settings: SourceProductName=Simulink  SourceProductBaseCode=SL
  cfblk15 : Delay
  cfblk16 : Delay
  cfblk3 : DiscreteIntegrator  SampleTime=-1  OutDataTypeStr=double  ICPrevOutput=DiscIntNeverNeededParam  ICPrevScaledInput=DiscIntNeverNeededParam
  cfblk4 : DiscreteZeroPole  Poles=[0 0.5]  Gain=1  SampleTime=-1
  cfblk5 : DiscreteStateSpace  SampleTime=-1
  cfblk6 : DiscreteIntegrator  SampleTime=-1  OutDataTypeStr=double  ICPrevOutput=DiscIntNeverNeededParam  ICPrevScaledInput=DiscIntNeverNeededParam
  cfblk7 : simulink/Continuous/PID Controller  Controller=PID  TimeDomain=Discrete-time  SampleTime=-1  IntegratorMethod=Forward Euler  FilterMethod=Forward Euler  Form=Parallel  UseFilter=on  ControllerParametersSource=internal  P=1  I=1  D=0  N=100  InitialConditionSource=internal  InitialConditionForIntegrator=0  InitialConditionForFilter=0  ExternalReset=none  LimitOutput=off  UpperSaturationLimit=inf  LowerSaturationLimit=-inf  LinearizeAsGain=off  AntiWindupMode=none  Kb=1  TrackingMode=off  Kt=1  PParamMin=[]  PParamMax=[]  IParamMin=[]  IParamMax=[]  DParamMin=[]  DParamMax=[]  NParamMin=[]  NParamMax=[]  KbParamMin=[]  KbParamMax=[]  KtParamMin=[]  KtParamMax=[]  POutMin=[]  POutMax=[]  IOutMin=[]  IOutMax=[]  DOutMin=[]  DOutMax=[]  NOutMin=[]  NOutMax=[]  KbOutMin=[]  KbOutMax=[]  KtOutMin=[]  KtOutMax=[]  IntegratorOutMin=[]  IntegratorOutMax=[]  FilterOutMin=[]  FilterOutMax=[]  SumOutMin=[]  SumOutMax=[]  SumI1OutMin=[]  SumI1OutMax=[]  SumI2OutMin=[]  SumI2OutMax=[]  SumI3OutMin=[]  SumI3OutMax=[]  SumDOutMin=[]  SumDOutMax=[]  SaturationOutMin=[]  SaturationOutMax=[]  IntegratorContinuousStateAttributes=''  IntegratorStateMustResolveToSignalObject=off  IntegratorRTWStateStorageClass=Auto  FilterContinuousStateAttributes=''  FilterStateMustResolveToSignalObject=off  FilterRTWStateStorageClass=Auto  DifferentiatorICPrevScaledInput=0  DifferentiatorOutMin=[]  DifferentiatorOutMax=[]  FilterDiffOutCoefMin=[]  FilterDiffOutCoefMax=[]  SumDenOutMin=[]  SumDenOutMax=[]  SumNumOutMin=[]  SumNumOutMax=[]  ReciprocalOutMin=[]  ReciprocalOutMax=[]  DivideOutMin=[]  DivideOutMax=[]  TunerSelectOption=Transfer Function Based (PID Tuner App)
  cfblk8 : Delay  DelayLengthSource=Input port
      settings: InputPortMap=u0,p1
  cfblk9 : Delay  ShowEnablePort=on
      settings: InputPortMap=u0,e6
  cyemi_{128..143} (16 alike) : DataTypeConversion  OutDataTypeStr=double
  cfblk2 : Outport
  cfblk14 : Outport  Port=2
  wires:
  cfblk9/1 -> cyemi_132/1, cyemi_139/1
  cfblk12/1 -> cfblk14/1, cyemi_133/1
  cfblk8/1 -> cyemi_128/1, cyemi_143/1
  cfblk1/1 -> cfblk2/1
  cfblk4/1 -> cyemi_137/1, cyemi_141/1
  cyemi_128/1 -> cfblk10/1
  cyemi_129/1 -> cfblk11/1
  cfblk6/1 -> cyemi_129/1
  cyemi_130/1 -> cfblk12/1
  cfblk13/1 -> cyemi_130/1
  cyemi_131/1 -> cfblk12/2
  cfblk11/1 -> cyemi_131/1
  cyemi_132/1 -> cfblk13/1
  cyemi_133/1 -> cfblk15/1
  cyemi_134/1 -> cfblk16/1
  cfblk5/1 -> cyemi_134/1
  cyemi_135/1 -> cfblk3/1
  cfblk15/1 -> cyemi_135/1
  cyemi_136/1 -> cfblk4/1
  cfblk16/1 -> cyemi_136/1
  cyemi_137/1 -> cfblk5/1
  cyemi_138/1 -> cfblk6/1
  cfblk7/1 -> cyemi_138/1
  cyemi_139/1 -> cfblk7/1
  cyemi_140/1 -> cfblk8/1
  cfblk3/1 -> cyemi_140/1
  cyemi_141/1 -> cfblk8/2
  cyemi_142/1 -> cfblk9/1
  cfblk10/1 -> cyemi_142/1
  cyemi_143/1 -> cfblk9/2

== system sampleModel7424_pp/cfblk126/cfblk12 ==
  cfblk1 : Inport
  cfblk10 : Inport  Port=2
  cfblk11 : Inport  Port=3
  cfblk12 : Inport  Port=4
  cfblk13 : Inport  Port=5
  Action Port : ActionPort  ActionType=then
  cfblk3 : DiscreteIntegrator  SampleTime=-1  OutDataTypeStr=double  ICPrevOutput=DiscIntNeverNeededParam  ICPrevScaledInput=DiscIntNeverNeededParam
  cfblk4 : simulink/Discrete/Transfer Fcn Real Zero  ZeroZ=0.75  ICPrevInput=0.0  DoSatur=off
      settings: SourceProductName=Simulink  SourceProductBaseCode=SL
  cfblk5 : simulink/Discrete/Difference  ICPrevInput=0.0  OutMin=[]  OutMax=[]  OutDataTypeStr=double  OutputDataTypeScalingMode=double  OutDataType=fixdt(1, 16)  OutScaling=2^-10  DoSatur=off
  cfblk6 : simulink/Discrete/Difference  ICPrevInput=0.0  OutMin=[]  OutMax=[]  OutDataTypeStr=double  OutputDataTypeScalingMode=double  OutDataType=fixdt(1, 16)  OutScaling=2^-10  DoSatur=off
  cfblk7 : DiscreteZeroPole  Poles=[0 0.5]  Gain=1  SampleTime=-1
  cfblk8 : simulink/Discrete/Transfer Fcn Real Zero  ZeroZ=0.75  ICPrevInput=0.0  DoSatur=off
      settings: SourceProductName=Simulink  SourceProductBaseCode=SL
  cfblk9 : simulink/Discrete/Transfer Fcn Real Zero  ZeroZ=0.75  ICPrevInput=0.0  DoSatur=off
      settings: SourceProductName=Simulink  SourceProductBaseCode=SL
  cyemi_{161..167} (7 alike) : DataTypeConversion  OutDataTypeStr=double
  cfblk2 : Outport
  cfblk14 : Outport  Port=2
  cfblk15 : Outport  Port=3
  wires:
  cfblk4/1 -> cfblk14/1
  cfblk7/1 -> cfblk15/1
  cfblk5/1 -> cfblk2/1
  cyemi_161/1 -> cfblk3/1
  cfblk10/1 -> cyemi_161/1
  cyemi_162/1 -> cfblk4/1
  cfblk13/1 -> cyemi_162/1
  cyemi_163/1 -> cfblk5/1
  cfblk9/1 -> cyemi_163/1
  cyemi_164/1 -> cfblk6/1
  cfblk3/1 -> cyemi_164/1
  cyemi_165/1 -> cfblk7/1
  cfblk11/1 -> cyemi_165/1
  cyemi_166/1 -> cfblk8/1
  cfblk6/1 -> cyemi_166/1
  cyemi_167/1 -> cfblk9/1
  cfblk1/1 -> cyemi_167/1

== system sampleModel7424_pp/cfblk126/cfblk13 ==
  cfblk1 : Inport
  Action Port : ActionPort  ActionType=else
  cfblk3 : DiscreteStateSpace  SampleTime=-1
  cfblk4 : simulink/Continuous/PID Controller  Controller=PID  TimeDomain=Discrete-time  SampleTime=-1  IntegratorMethod=Forward Euler  FilterMethod=Forward Euler  Form=Parallel  UseFilter=on  ControllerParametersSource=internal  P=1  I=1  D=0  N=100  InitialConditionSource=internal  InitialConditionForIntegrator=0  InitialConditionForFilter=0  ExternalReset=none  LimitOutput=off  UpperSaturationLimit=inf  LowerSaturationLimit=-inf  LinearizeAsGain=off  AntiWindupMode=none  Kb=1  TrackingMode=off  Kt=1  PParamMin=[]  PParamMax=[]  IParamMin=[]  IParamMax=[]  DParamMin=[]  DParamMax=[]  NParamMin=[]  NParamMax=[]  KbParamMin=[]  KbParamMax=[]  KtParamMin=[]  KtParamMax=[]  POutMin=[]  POutMax=[]  IOutMin=[]  IOutMax=[]  DOutMin=[]  DOutMax=[]  NOutMin=[]  NOutMax=[]  KbOutMin=[]  KbOutMax=[]  KtOutMin=[]  KtOutMax=[]  IntegratorOutMin=[]  IntegratorOutMax=[]  FilterOutMin=[]  FilterOutMax=[]  SumOutMin=[]  SumOutMax=[]  SumI1OutMin=[]  SumI1OutMax=[]  SumI2OutMin=[]  SumI2OutMax=[]  SumI3OutMin=[]  SumI3OutMax=[]  SumDOutMin=[]  SumDOutMax=[]  SaturationOutMin=[]  SaturationOutMax=[]  IntegratorContinuousStateAttributes=''  IntegratorStateMustResolveToSignalObject=off  IntegratorRTWStateStorageClass=Auto  FilterContinuousStateAttributes=''  FilterStateMustResolveToSignalObject=off  FilterRTWStateStorageClass=Auto  DifferentiatorICPrevScaledInput=0  DifferentiatorOutMin=[]  DifferentiatorOutMax=[]  FilterDiffOutCoefMin=[]  FilterDiffOutCoefMax=[]  SumDenOutMin=[]  SumDenOutMax=[]  SumNumOutMin=[]  SumNumOutMax=[]  ReciprocalOutMin=[]  ReciprocalOutMax=[]  DivideOutMin=[]  DivideOutMax=[]  TunerSelectOption=Transfer Function Based (PID Tuner App)
  cfblk5 : simulink/Continuous/PID Controller (2DOF)  Controller=PID  TimeDomain=Discrete-time  SampleTime=-1  IntegratorMethod=Forward Euler  FilterMethod=Forward Euler  Form=Parallel  UseFilter=on  ControllerParametersSource=internal  P=1  I=1  D=0  N=100  b=1  c=1  InitialConditionSource=internal  InitialConditionForIntegrator=0  InitialConditionForFilter=0  ExternalReset=none  LimitOutput=off  UpperSaturationLimit=inf  LowerSaturationLimit=-inf  LinearizeAsGain=off  AntiWindupMode=none  Kb=1  TrackingMode=off  Kt=1  PParamMin=[]  PParamMax=[]  IParamMin=[]  IParamMax=[]  DParamMin=[]  DParamMax=[]  NParamMin=[]  NParamMax=[]  bParamMin=[]  bParamMax=[]  cParamMin=[]  cParamMax=[]  KbParamMin=[]  KbParamMax=[]  KtParamMin=[]  KtParamMax=[]  POutMin=[]  POutMax=[]  IOutMin=[]  IOutMax=[]  DOutMin=[]  DOutMax=[]  NOutMin=[]  NOutMax=[]  bOutMin=[]  bOutMax=[]  cOutMin=[]  cOutMax=[]  KbOutMin=[]  KbOutMax=[]  KtOutMin=[]  KtOutMax=[]  IntegratorOutMin=[]  IntegratorOutMax=[]  FilterOutMin=[]  FilterOutMax=[]  SumOutMin=[]  SumOutMax=[]  Sum1OutMin=[]  Sum1OutMax=[]  Sum2OutMin=[]  Sum2OutMax=[]  Sum3OutMin=[]  Sum3OutMax=[]  SumI1OutMin=[]  SumI1OutMax=[]  SumI2OutMin=[]  SumI2OutMax=[]  SumI3OutMin=[]  SumI3OutMax=[]  SumDOutMin=[]  SumDOutMax=[]  SaturationOutMin=[]  SaturationOutMax=[]  IntegratorContinuousStateAttributes=''  IntegratorStateMustResolveToSignalObject=off  IntegratorRTWStateStorageClass=Auto  FilterContinuousStateAttributes=''  FilterStateMustResolveToSignalObject=off  FilterRTWStateStorageClass=Auto  DifferentiatorICPrevScaledInput=0  DifferentiatorOutMin=[]  DifferentiatorOutMax=[]  FilterDiffOutCoefMin=[]  FilterDiffOutCoefMax=[]  SumDenOutMin=[]  SumDenOutMax=[]  SumNumOutMin=[]  SumNumOutMax=[]  ReciprocalOutMin=[]  ReciprocalOutMax=[]  DivideOutMin=[]  DivideOutMax=[]  TunerSelectOption=Transfer Function Based (PID Tuner App)
  cfblk6 : simulink/Discrete/Transfer Fcn First Order  PoleZ=0.95  ICPrevOutput=0.0  DoSatur=off
      settings: SourceProductName=Simulink
  cfblk8 : Delay
  cyemi_{169..174} (6 alike) : DataTypeConversion  OutDataTypeStr=double
  cfblk2 : Outport
  cfblk7 : Outport  Port=2
  wires:
  cfblk4/1 -> cfblk2/1, cfblk7/1
  cfblk6/1 -> cyemi_170/1, cyemi_174/1
  cyemi_169/1 -> cfblk3/1
  cfblk5/1 -> cyemi_169/1
  cyemi_170/1 -> cfblk4/1
  cyemi_171/1 -> cfblk5/1
  cfblk1/1 -> cyemi_171/1
  cyemi_172/1 -> cfblk5/2
  cfblk8/1 -> cyemi_172/1
  cyemi_173/1 -> cfblk6/1
  cfblk3/1 -> cyemi_173/1
  cyemi_174/1 -> cfblk8/1
